simulink model "model_sys"  (R2024a)
settings: Solver=FixedStepDiscrete  StartTime=0.0  StopTime=Tf  FixedStep=Ts  RelTol=1e-3
model workspace (MAT data in the model file):
  I_ref = 6.5
  Ki_torque = 36
  Kp_torque = 0.04
  T_save_start = 0.3
  Tf = 0.5
  Ts = 1e-06
  capacitor_C = 0.000332
  capacitor_R = 0.03
  freq_ref = 60
  fsw = 100000
  source_L = 0
  source_R = 0
libraries: spsThreePhaseVIMeasurementLib x3, spsSeriesRLCBranchLib x2, spsThreePhaseSourceLib x1, spsThreePhaseTransformerTwoWindingsLib x1, spsAsynchronousMachineSIUnitsLib x1, spsTwoLevelConverterLib x1, spsMultimeterLib x1, spsPWMGenerator2LevelLib x1, spsUniversalBridgeLib x1, slpidlib x1, spsRMSLib x1, spspowerguiLib x1
settings Model: SimulationMode=accelerator  Creator=thalerg  LastModifiedBy=thalerg
settings DataIOCC: SaveOutput=off  DSMLogging=off  SaveTime=off  LoggingIntervals=[T_save_start, inf]
settings ModelReferenceCC: UpdateModelReferenceTargets=IfOutOfDate  EnableRefExpFcnMdlSchedulingChecks=on
settings CodeAppCC: StateflowObjectComments=on
settings ConfigComp: CovExternalEMLEnable=off
settings SimscapeCC: SimscapeNormalizeSystem=off

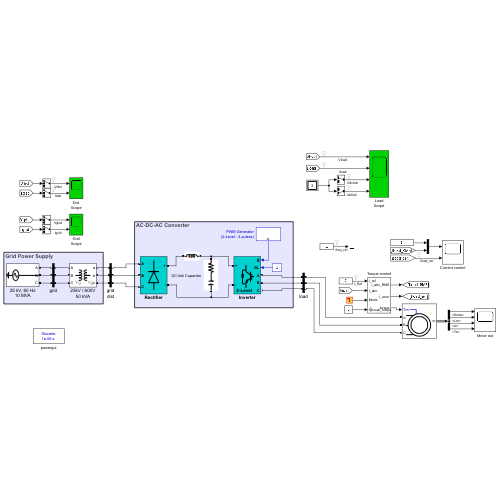
[thumbnail: Simulink's stored preview of the top-level diagram]
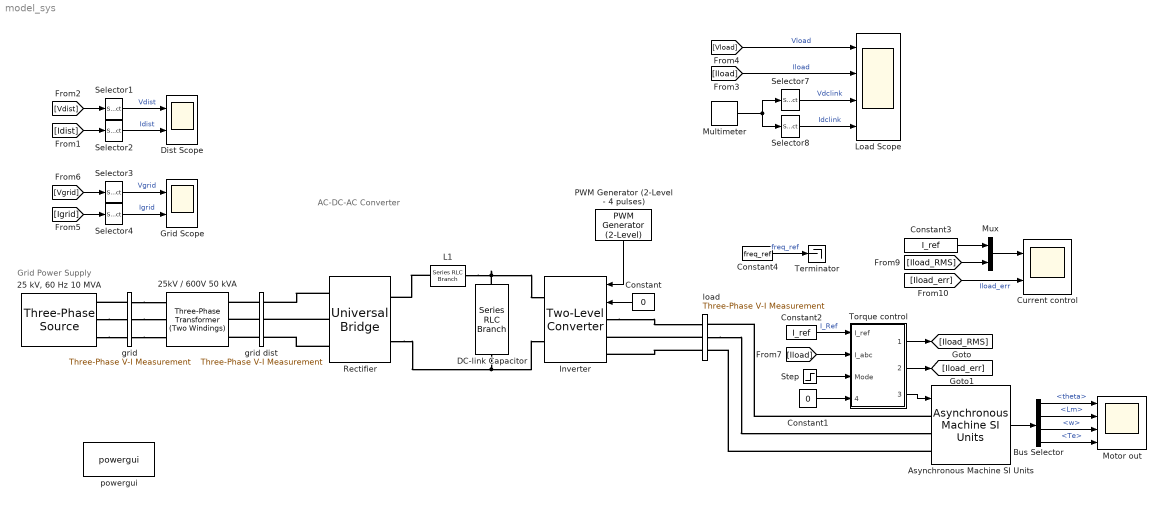
== system model_sys ==
  note: Grid Power Supply
  note: AC-DC-AC Converter
  "25 kV, 60 Hz 10 MVA" : spsThreePhaseSourceLib/Three-Phase Source  InternalConnection=Yg  VoltagePhases=off  Voltage=25e3  PhaseAngle=0  Voltage_phases=[25e3 25e3 25e3]/sqrt(3)  PhaseAngles_phases=[0 -120 +120]  Frequency=60  NonIdealSource=on  SpecifyImpedance=off  Resistance=source_R  Inductance=source_L  ShortCircuitLevel=10e6  BaseVoltage=25e3  XRratio=5  BusType=swing  Pref=0  Qref=0  Prefabc=[10e3, 10e3, 10e3]  Qrefabc=[0, 0, 0]  Qmin=-inf  Qmax=inf
  25kV / 600V 50 kVA : spsThreePhaseTransformerTwoWindingsLib/Three-Phase Transformer (Two Windings)  Winding1Connection=Yg  Winding2Connection=Yg  CoreType=Three single-phase transformers  SetSaturation=off  Hysteresis=off  DataFile='hysteresis'  SetInitialFlux=off  Measurements=None  UNITS=pu  NominalPower=[ 50e3 , 60 ]  Winding1=[ 25e3 , 0.004 , 0.02 ]  Winding2=[ 220*sqrt(3) , 0.004 , 0.02 ]  Rm=200  Lm=200  L0=0.5  Saturation="[ 0,0  ;  0.005,1.2  ;  1.0,1.4 ]"  InitialFluxes=[ 0.8 , -0.8 , 0.7 ]  BreakLoop=off  DiscreteSolver=Trapezoidal iterative  DataType=off  TransfoNumber=0
  Asynchronous Machine SI Units : spsAsynchronousMachineSIUnitsLib/Asynchronous Machine SI Units  RotorType=Squirrel-cage  PresetModel=No  MechanicalLoad=Torque Tm  ShowDetailedParameters=on  ReferenceFrame=Rotor  Units=SI  MeasurementBus=on  NominalParameters=[3000 380 60]  VoltageRatio=1  Stator=[0.6837 0.004152]  Rotor=[0.451 0.004152]  Cage1=[0.4155 0.002066]  Cage2=[0.4168 0.0003495]  Lm=0.1486  Mechanical=[0.0120 0.008141 2]  PolePairs=2  InitialConditions=[0 0 0 0 0 0 0 0]  SimulateSaturation=off  Saturation=[14.03593122, 27.81365428, 53.79336849, 72.68890987, 97.98006896, 148.6815601, 215.7428561, 302.9841135, 428.7778367 ; 230, 322, 414, 460, 506, 552, 598, 644, 690]  LoadFlowParameters=1492000  TsPowergui=0  TsBlock=-1  IterativeModel=Trapezoidal non iterative  IterativeDiscreteModel=Trapezoidal non iterative  Pmec=1.492e+006
  Bus Selector : BusSelector  OutputSignals=theta,Lm,w,Te
  Constant : Constant  Value=0
  Constant1 : Constant  Value=0  SampleTime=Ts
  Constant2 : Constant  Value=I_ref  SampleTime=Ts
  Constant3 : Constant  Value=I_ref  SampleTime=Ts
  Constant4 : Constant  Value=freq_ref  SampleTime=Ts
  Current control : Scope  NumInputPorts=2
  DC-link Capacitor : spsSeriesRLCBranchLib/Series RLC Branch  LConnTagsString=__new0  RConnTagsString=__new0  BranchType=RC  Resistance=capacitor_R  Inductance=1e-3  SetiL0=off  InitialCurrent=0  Capacitance=capacitor_C  Setx0=on  InitialVoltage=500  Measurements=Branch voltage and current
  Dist Scope : Scope  NumInputPorts=2
  Grid Scope : Scope  NumInputPorts=2
  Inverter : spsTwoLevelConverterLib/Two-Level Converter  ModelType=Switching devices  Ron=1e-3  Rs=1e6  Cs=inf  Vforward=[0,0]  Ron_Diode=1e-3  Rs_Diode=1e6  Cs_Diode=inf  Vf_Diode=1e-3  Rs_CurrentSource=inf  Ron_ACsource=1e-3
      settings: LibrarySourceBlock=sps_lib/Power Electronics/Two-Level Converter
  L1 : spsSeriesRLCBranchLib/Series RLC Branch  LConnTagsString=__new0  RConnTagsString=__new0  BranchType=L  Resistance=1.0  Inductance=200e-6  SetiL0=off  InitialCurrent=0  Capacitance=1.0  Setx0=off  InitialVoltage=0  Measurements=None
  Load Scope : Scope  NumInputPorts=4
  Motor out : Scope  NumInputPorts=4
  Multimeter : spsMultimeterLib/Multimeter  L=2  sel=[1 2]  yselected={}  Gain=[1 1]  OutputType=Complex  PlotAtSimulationStop=off  PhasorSimulation=off
  Mux : Mux  Inputs=2
  PWM Generator (2-Level - 4 pulses) : spsPWMGenerator2LevelLib/PWM Generator (2-Level)  ModulatorType=Three-phase bridge (6 pulses)  ModulatorMode=Unsynchronized  Fc=fsw  Pc=90  nF=27  MinMax="[ -1  1 ]"  SamplingTechnique=Natural  ModulatingSignals=on  m=0.8  Freq=freq_ref  Phase=0  Ts=Ts  ShowCarrierOutport=off
  Rectifier : spsUniversalBridgeLib/Universal Bridge  Arms=3  SnubberResistance=100  SnubberCapacitance=0.1e-6  Device=Diodes  Ron=1e-3  Lon=0  ForwardVoltages="[  0.8  0.8  ]"  ForwardVoltage=.8  GTOparameters=[ 10e-6 , 20e-6 ]  IGBTparameters=[ 1e-6 , 2e-6 ]  Measurements=None  Measurements_2=None  converterType=Rectifier
      settings: AttributesFormatString=\n
  Selector{1..4} (4 alike) : Selector  IndexMode=Zero-based  InputPortWidth=3  IndexOptions=Index vector (dialog)  Indices=0  OutputSizes=1
  Selector7 : Selector  IndexMode=Zero-based  InputPortWidth=2  IndexOptions=Index vector (dialog)  Indices=0  OutputSizes=1
  Selector8 : Selector  IndexMode=Zero-based  InputPortWidth=2  IndexOptions=Index vector (dialog)  Indices=1  OutputSizes=1
  Step : Step  Time=0.1  Before=1  After=0  SampleTime=Ts
  Terminator : Terminator
  Torque control : Subsystem  mask(PI Torque control){Kp=Kp_torque, Ki=Ki_torque}
      mask help: Simple PI for motor torque control. Reference is the desired RMS current, process variable is the load current.
  grid : spsThreePhaseVIMeasurementLib/Three-Phase V-I Measurement  VoltageMeasurement=phase-to-ground  SetLabelV=on  LabelV=Vgrid  Vpu=off  VpuLL=off  CurrentMeasurement=yes  SetLabelI=on  LabelI=Igrid  Ipu=off  Pbase=1e3  Vbase=380  OutputType=Magnitude  PhasorSimulation=off  PSBequivalent=0
  grid dist : spsThreePhaseVIMeasurementLib/Three-Phase V-I Measurement  VoltageMeasurement=phase-to-ground  SetLabelV=on  LabelV=Vdist  Vpu=off  VpuLL=off  CurrentMeasurement=yes  SetLabelI=on  LabelI=Idist  Ipu=off  Pbase=1e3  Vbase=380  OutputType=Magnitude  PhasorSimulation=off  PSBequivalent=0
  load : spsThreePhaseVIMeasurementLib/Three-Phase V-I Measurement  VoltageMeasurement=phase-to-ground  SetLabelV=on  LabelV=Vload  Vpu=off  VpuLL=off  CurrentMeasurement=yes  SetLabelI=on  LabelI=Iload  Ipu=off  Pbase=1e3  Vbase=380  OutputType=Magnitude  PhasorSimulation=off  PSBequivalent=0
  powergui : spspowerguiLib/powergui  Priority=1  SimulationMode=Discrete  SampleTime=Ts  frequency=60  Iterations=50  frequencyindice=60  Pbase=100e6  ErrMax=1e-4  UnitsV=kV  UnitsW=MW  buscounter=0  FunctionMessages=off  echomessages=off  EnableUseOfTLC=off  CurrentSourceSwitches=off  DisableSnubberDevices=off  DisableRonSwitches=off  DisableVfSwitches=off  DisplayEquations=off  AutomaticDiscreteSolvers=off  SolverType=Tustin/Backward Euler (TBE)  Interpol=off  ExternalGateDelay=off  methode=off  Ts=100  x0status=blocks  SPID=off  SwTol=0  HookPort=off  NonlinearTolerance=1e-4  nMaxIteration=100  ContinueOnMaxIteration=off  RestoreLinks=warning  ResistiveCurrentMeasurement=off  Frange=[0:2:500]  Ylog=off  Xlog=on  ShowGrid=off  save=off  variable=ZData  structure=0  ZoomFFT=off  StartTime=0.0  cycles=1  DisplayStyle=1  fundamental=60  FreqAxis=off  MaxFrequency=1000  frequencyindicesteady=1  RmsSteady=1  display=off
  wires:
  Selector4/1 -> Grid Scope/2  "Igrid"
  Selector3/1 -> Grid Scope/1  "Vgrid"
  [Igrid] -> Selector4/1
  [Vgrid] -> Selector3/1
  [Vdist] -> Selector1/1
  [Idist] -> Selector2/1
  Selector1/1 -> Dist Scope/1  "Vdist"
  Selector2/1 -> Dist Scope/2  "Idist"
  PWM Generator (2-Level - 4 pulses)/1 -> Inverter/1
  Constant/1 -> Inverter/2
  Multimeter/1 -> Selector8/1, Selector7/1
  [Vload] -> Load Scope/1  "Vload"
  [Iload] -> Load Scope/2  "Iload"
  Bus Selector/4 -> Motor out/4  "<Te>"
  Constant1/1 -> Torque control/4(Manual_torque)
  Bus Selector/1 -> Motor out/1  "<theta>"
  Bus Selector/3 -> Motor out/3  "<w>"
  Torque control/3(torque) -> Asynchronous Machine SI Units/1
  Step/1 -> Torque control/3(Mode)
  Bus Selector/2 -> Motor out/2  "<Lm>"
  Asynchronous Machine SI Units/1 -> Bus Selector/1
  Selector7/1 -> Load Scope/3  "Vdclink"
  Selector8/1 -> Load Scope/4  "Idclink"
  [Iload] -> Torque control/2(I_abc)
  Constant2/1 -> Torque control/1(I_ref)  "I_Ref"
  Torque control/1(I_abc_RMS) -> [Iload_RMS]
  Torque control/2(I_error) -> [Iload_err]
  Mux/1 -> Current control/1
  Constant3/1 -> Mux/1
  [Iload_RMS] -> Mux/2
  [Iload_err] -> Current control/2  "Iload_err"
  Constant4/1 -> Terminator/1  "freq_ref"
  connections:
  "25 kV, 60 Hz 10 MVA"/RConn3 -- grid/LConn3
  grid/LConn1 -- "25 kV, 60 Hz 10 MVA"/RConn1
  grid/RConn1 -- 25kV / 600V 50 kVA/LConn1
  "25 kV, 60 Hz 10 MVA"/RConn2 -- grid/LConn2
  grid/RConn2 -- 25kV / 600V 50 kVA/LConn2
  grid/RConn3 -- 25kV / 600V 50 kVA/LConn3
  grid dist/LConn1 -- 25kV / 600V 50 kVA/RConn1
  grid dist/LConn2 -- 25kV / 600V 50 kVA/RConn2
  grid dist/LConn3 -- 25kV / 600V 50 kVA/RConn3
  DC-link Capacitor/LConn1 -- L1/RConn1 -- Inverter/RConn1
  Inverter/RConn2 -- Rectifier/RConn2 -- DC-link Capacitor/RConn1
  load/LConn3 -- Inverter/LConn3
  Inverter/LConn1 -- load/LConn1
  Rectifier/LConn2 -- grid dist/RConn2
  Rectifier/LConn3 -- grid dist/RConn3
  L1/LConn1 -- Rectifier/RConn1
  load/LConn2 -- Inverter/LConn2
  Rectifier/LConn1 -- grid dist/RConn1
  Asynchronous Machine SI Units/LConn1 -- load/RConn1
  load/RConn2 -- Asynchronous Machine SI Units/LConn2
  Asynchronous Machine SI Units/LConn3 -- load/RConn3

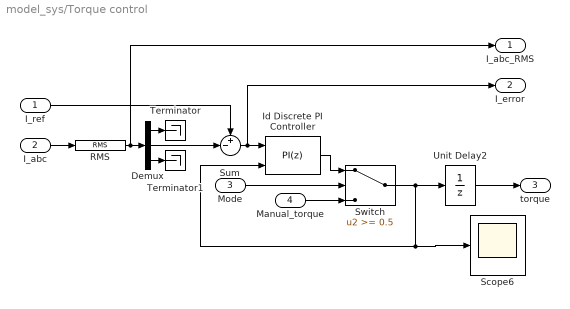
== system model_sys/Torque control ==
  I_ref : Inport
  I_abc : Inport  Port=2
  Mode : Inport  Port=3
  Manual_torque : Inport  Port=4
  Demux : Demux  Outputs=3
  Id Discrete PI Controller : slpidlib/PID Controller  Controller=PI  Form=Parallel  TimeDomain=Discrete-time  UseExternalTs=off  SampleTime=Ts  IntegratorMethod=Forward Euler  FilterMethod=Forward Euler  ControllerParametersSource=internal  P=Kp_torque  I=Ki_torque  UseKiTs=off  D=0  UseExternalDerivativeSource=off  N=100  UseFilter=on  TunerSelectOption=Transfer Function Based (PID Tuner App)  InitialConditionSource=internal  InitialConditionForIntegrator=0.5  InitialConditionForFilter=0  DifferentiatorICPrevScaledInput=0  ExternalReset=none  TrackingMode=on  Kt=1  LimitOutput=on  SatLimitsSource=internal  UpperSaturationLimit=inf  LowerSaturationLimit=0  LinearizeAsGain=off  AntiWindupMode=clamping  Kb=1  LimitIntegrator=off  UpperIntegratorSaturationLimit=inf  LowerIntegratorSaturationLimit=-inf  POutMin=[]  POutMax=[]  IOutMin=[]  IOutMax=[]  DOutMin=[]  DOutMax=[]  NOutMin=[]  NOutMax=[]  SumOutMin=[]  SumOutMax=[]  SaturationOutMin=[]  SaturationOutMax=[]  PParamMin=[]  PParamMax=[]  IParamMin=[]  IParamMax=[]  DParamMin=[]  DParamMax=[]  NParamMin=[]  NParamMax=[]  KbParamMin=[]  KbParamMax=[]  KtParamMin=[]  KtParamMax=[]  KbOutMin=[]  KbOutMax=[]  KtOutMin=[]  KtOutMax=[]  IntegratorOutMin=[]  IntegratorOutMax=[]  FilterOutMin=[]  FilterOutMax=[]  SumI1OutMin=[]  SumI1OutMax=[]  SumI2OutMin=[]  SumI2OutMax=[]  SumI3OutMin=[]  SumI3OutMax=[]  SumI4OutMin=[]  SumI4OutMax=[]  SumDOutMin=[]  SumDOutMax=[]  DifferentiatorOutMin=[]  DifferentiatorOutMax=[]  FilterDiffOutCoefMin=[]  FilterDiffOutCoefMax=[]  ReciprocalOutMin=[]  ReciprocalOutMax=[]  SumDenOutMin=[]  SumDenOutMax=[]  SumNumOutMin=[]  SumNumOutMax=[]  DivideOutMin=[]  DivideOutMax=[]  UdiffTsProdOutMin=[]  UdiffTsProdOutMax=[]  NTsProdOutMin=[]  NTsProdOutMax=[]  UintegralTsProdOutMin=[]  UintegralTsProdOutMax=[]  UngainTsProdOutMin=[]  UngainTsProdOutMax=[]  ClampingZeroOutDataTypeStr=Inherit: Inherit via back propagation  ClampingZeroOutMin=[]  ClampingZeroOutMax=[]  FilterDenConstantOutDataTypeStr=Inherit: Inherit via back propagation  FilterDenConstantOutMin=[]  FilterDenConstantOutMax=[]  PCopyOutDataTypeStr=Inherit: Inherit via back propagation  PCopyOutMin=[]  PCopyOutMax=[]  NCopyOutDataTypeStr=Inherit: Inherit via back propagation  NCopyOutMin=[]  NCopyOutMax=[]  IntegratorContinuousStateAttributes=''  IntegratorStateMustResolveToSignalObject=off  IntegratorRTWStateStorageClass=Auto  FilterContinuousStateAttributes=''  FilterStateMustResolveToSignalObject=off  FilterRTWStateStorageClass=Auto  ParallelPVariant=InternalParameters  IdealPVariant=Disabled  IVariant=InternalParameters  DVariant=Disabled  IntegratorVariant=Discrete  SatVariant=Enabled  AWVariant=DiscClampingParallel  PCopyVariant=Disabled  TRVariant=Enabled  FdbkBlocksVariant=Forward  IdealPFdbkVariant=Disabled  SatFdbkVariant=Disabled  DerivativeFilterVariant=Disabled  NVariant=Disabled  NCopyVariant=Disabled_SignalSpec  FilterICVariant=Disabled  IntegratorICVariant=InternalICs  ExternalResetVariant=Disabled  TRSumVariant=TrackingMode  SumFdbkVariant=Disabled  SumVariant=Sum_PI  TsampFilterVariant=InternalTs  TsampNgainVariant=Passthrough  TsampIntegralVariant=Disabled_SignalSpec  ExternalSaturationOutDataTypeStr=Inherit: Same as second input  DerivativeSourceVariant=Disabled
  RMS : spsRMSLib/RMS  TrueRMS=on  Freq=freq_ref  RMSInit=0  Ts=Ts
  Scope6 : Scope
  Sum : Sum  Inputs=+-|
  Switch : Switch  Threshold=0.5  SaturateOnIntegerOverflow=off  InputSameDT=off
  Terminator : Terminator
  Terminator1 : Terminator
  Unit Delay2 : UnitDelay  SampleTime=-1  HasFrameUpgradeWarning=on
  I_abc_RMS : Outport
  I_error : Outport  Port=2
  torque : Outport  Port=3
  wires:
  Unit Delay2/1 -> torque/1
  Sum/1 -> I_error/1, Id Discrete PI Controller/1
  I_abc/1 -> RMS/1
  I_ref/1 -> Sum/1
  RMS/1 -> I_abc_RMS/1, Demux/1
  Demux/2 -> Sum/2
  Switch/1 -> Scope6/1, Id Discrete PI Controller/2, Unit Delay2/1
  Id Discrete PI Controller/1 -> Switch/1
  Mode/1 -> Switch/2
  Manual_torque/1 -> Switch/3
  Demux/1 -> Terminator/1
  Demux/3 -> Terminator1/1
